simulink model "Bixler"  (R2018b)
settings: Solver=FixedStepAuto  StartTime=0.0  StopTime=inf  RelTol=1e-3
undefined symbols (not defined in the file or in its folder): dev, Main, pwm_output0
libraries: px4uORBlib x3, px4Sensorslib x2, simulink x2, px4lib x1, sharedtransform x1
settings Model: SimulationMode=external  ExtModeTrigDuration=10  Creator=Robert  LastModifiedBy=Robert
settings SolverCC: PositivePriorityOrder=on
settings OptimizationCC: EnhancedBackFolding=on  PassReuseOutputArgsAs=Individual arguments  MaxStackSize=64  OptimizeBlockOrder=speed  DifferentSizesBufferReuse=on  OptimizationCustomize=off
settings DebuggingCC: ParameterTunabilityLossMsg=error
settings HardwareCC: ProdBitPerPointer=32  ProdBitPerSizeT=32  ProdBitPerPtrDiffT=32  ProdLargestAtomicInteger=Long  ProdLargestAtomicFloat=Double  ProdWordSize=32  ProdLongLongMode=on  ProdHWDeviceType=ARM Compatible->ARM Cortex
settings SFSimCC: MATLABDynamicMemAlloc=off
settings RTWCC: SystemTargetFile=ert.tlc  HardwareBoard=PX4 Pixhawk 1  TLCOptions="-aInlineSetEventsForThisBaseRateFcn=TLC_FALSE -aSuppressMultiTaskScheduler=TLC_FALSE  -aRateBasedStepFcn=0"  TemplateMakefile=ert_default_tmf  GenerateReport=on  Toolchain=GNU Tools for PX4 Autopilots  IncludeHyperlinkInReport=on  LaunchReport=on  TargetLang=C++  GenerateTraceInfo=on  GenerateTraceReport=on  GenerateTraceReportSl=on  GenerateTraceReportSf=on  GenerateTraceReportEml=on
settings CodeAppCC: ForceParamTrailComments=on  IgnoreCustomStorageClasses=off  OperatorAnnotations=on  SimulinkDataObjDesc=on  SFDataObjDesc=on  InsertBlockDesc=on
settings ERTTargetCC: ExtMode=on  ExtModeMexArgs='127.0.0.1' 1 17725

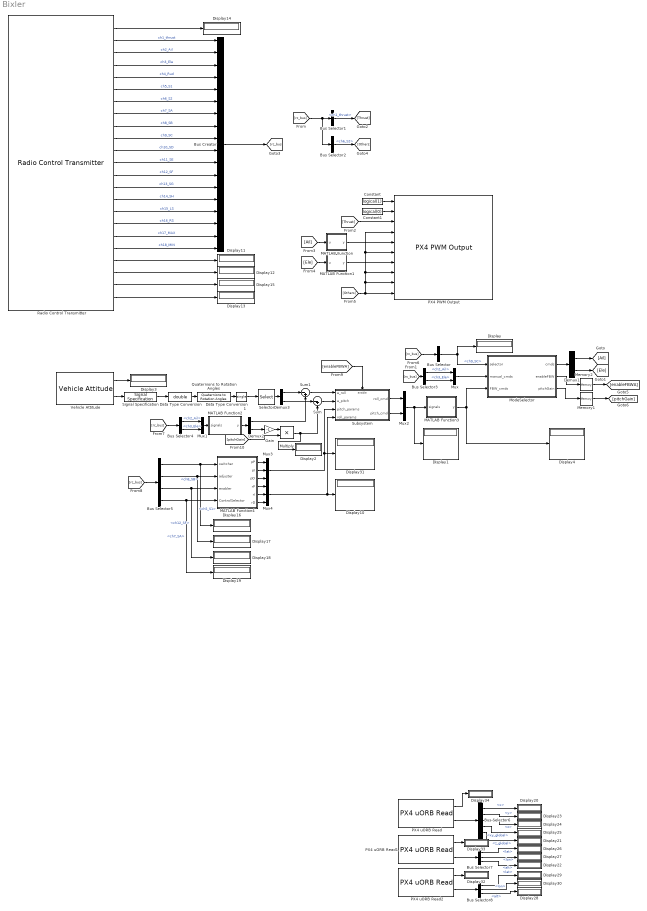
== system Bixler ==
  Bus Creator : BusCreator  Inputs=18
  Bus Selector : BusSelector  OutputSignals=ch9_SC
  Bus Selector1 : BusSelector  OutputSignals=ch1_thrust
  Bus Selector2 : BusSelector  OutputSignals=ch6_S2
  Bus Selector3 : BusSelector  OutputSignals=ch2_Ail,ch3_Ele
  Bus Selector4 : BusSelector  OutputSignals=ch2_Ail,ch3_Ele
  Bus Selector5 : BusSelector  OutputSignals=ch8_SB,ch5_S1,ch12_SF,ch7_SA
  Bus Selector6 : BusSelector  OutputSignals=x,y,z,xy_global,z_global
  Bus Selector7 : BusSelector  OutputSignals=lat,lon,alt
  Bus Selector8 : BusSelector  OutputSignals=lat,lon,alt
  Constant : Constant  Value=logical(1)
  Constant1 : Constant  Value=logical(0)
  Data Type Conversion : DataTypeConversion  OutDataTypeStr=double
  Data Type Conversion1 : DataTypeConversion  OutDataTypeStr=single
  Demux1 : Demux  Outputs=2
  Demux2 : Demux  Outputs=2
  Demux3 : Demux  Outputs=2
  Display{,1..4,10..34} (30 alike) : Display
  Gain : Gain  Gain=-1
  MATLAB Function : MATLAB Function  TreatAsAtomicUnit=on
  MATLAB Function1 : MATLAB Function  TreatAsAtomicUnit=on
  MATLAB Function2 : MATLAB Function  TreatAsAtomicUnit=on
  MATLAB Function3 : MATLAB Function  TreatAsAtomicUnit=on
  MATLAB Function4 : MATLAB Function  TreatAsAtomicUnit=on
  Memory1 : Memory
  Memory2 : Memory
  ModeSelector : MATLAB Function  TreatAsAtomicUnit=on
  Multiply : Product
  Mux : Mux  Inputs=2
  Mux1 : Mux  Inputs=2
  Mux2 : Mux  Inputs=2
  Mux3 : Mux  Inputs=3
  Mux4 : Mux  Inputs=3
  PX4 PWM Output : px4lib/PX4 PWM Output  pwmDevice=Main (/dev/pwm_output0)  pwmChannel1_=on  pwmChannel2_=on  pwmChannel3_=on  pwmChannel4_=on  pwmChannel5_=on  pwmChannel6_=on  pwmChannel7_=on  pwmChannel8_=on  forceTerminateFailsafe=off  outputErrorStatus=off
      settings: SourceProductName=Embedded Coder Support Package for PX4 Autopilots
  PX4 uORB Read : px4uORBlib/PX4 uORB Read  uORBTopic=vehicle_local_position  sampleTime=0.001  BlockingMode=off  BlockTimeout=1e-3
      settings: SourceProductName=Embedded Coder Support Package for PX4 Autopilots
  PX4 uORB Read1 : px4uORBlib/PX4 uORB Read  uORBTopic=vehicle_global_position  sampleTime=0.001  BlockingMode=off  BlockTimeout=1e-3
      settings: SourceProductName=Embedded Coder Support Package for PX4 Autopilots
  PX4 uORB Read2 : px4uORBlib/PX4 uORB Read  uORBTopic=vehicle_gps_position  sampleTime=0.001  BlockingMode=off  BlockTimeout=1e-3
      settings: SourceProductName=Embedded Coder Support Package for PX4 Autopilots
  Quaternions to Rotation Angles : sharedtransform/Quaternions to Rotation Angles  rotationOrder=ZYX  aMode=aMode
      settings: SourceProductBaseCode=AE
  Radio Control Transmitter : px4Sensorslib/Radio Control Transmitter  channel1=on  channel2=on  channel3=on  channel4=on  channel5=on  channel6=on  channel7=on  channel8=on  channel9=on  channel10=on  channel11=on  channel12=on  channel13=on  channel14=on  channel15=on  channel16=on  channel17=on  channel18=on  channel_count=on  rssi=on  rc_input_source=on  timestamp_last_signal=on  time_stamp=off  sampleTime=1/250  BlockingMode=off  BlockTimeout=5
      settings: SourceProductName=Embedded Coder Support Package for PX4 Autopilots
  Selector : Selector  InputPortWidth=3  IndexOptions=Index vector (dialog)  Indices=[3 2]  OutputSizes=1
  Signal Specification : SignalSpecification  OutDataTypeStr=single
  Subsystem : Subsystem
  Sum : Sum  Inputs=|-+
  Sum1 : Sum  Inputs=|-+
  Vehicle Attitude : px4Sensorslib/Vehicle Attitude  rollRate=off  pitchRate=off  yawRate=off  quaternion=on  uorbTimeStamp=off  BlockingMode=off  BlockTimeout=0.001  sampleTime=1/250
      settings: SourceProductName=Embedded Coder Support Package for PX4 Autopilots
  wires:
  Vehicle Attitude/2 -> Signal Specification/1
  Vehicle Attitude/1 -> Display3/1
  Radio Control Transmitter/8 -> Bus Creator/7  "ch7_SA"
  Radio Control Transmitter/7 -> Bus Creator/6  "ch6_S2"
  Radio Control Transmitter/6 -> Bus Creator/5  "ch5_S1"
  Radio Control Transmitter/2 -> Bus Creator/1  "ch1_thrust"
  Radio Control Transmitter/3 -> Bus Creator/2  "ch2_Ail"
  Radio Control Transmitter/4 -> Bus Creator/3  "ch3_Ele"
  Radio Control Transmitter/5 -> Bus Creator/4  "ch4_Rud"
  Radio Control Transmitter/9 -> Bus Creator/8  "ch8_SB"
  Radio Control Transmitter/20 -> Display11/1
  Radio Control Transmitter/21 -> Display12/1
  Radio Control Transmitter/23 -> Display13/1
  Radio Control Transmitter/1 -> Display14/1
  Radio Control Transmitter/22 -> Display15/1
  Constant/1 -> PX4 PWM Output/1
  Bus Selector1/1 -> [Thrust]  "<ch1_thrust>"
  [Others] -> PX4 PWM Output/6, PX4 PWM Output/4, PX4 PWM Output/8, PX4 PWM Output/9, PX4 PWM Output/10
  Constant1/1 -> PX4 PWM Output/2
  Bus Creator/1 -> [rc_bus]
  Quaternions to Rotation Angles/1 -> Data Type Conversion1/1
  Bus Selector/1 -> ModeSelector/1(selector), Display/1  "<ch9_SC>"
  Demux3/1 -> Sum1/1
  Demux3/2 -> Sum/1
  Mux2/1 -> Display1/1, MATLAB Function3/1(signals)
  Signal Specification/1 -> Data Type Conversion/1
  Data Type Conversion1/1 -> Selector/1
  [rc_bus] -> Bus Selector2/1, Bus Selector1/1
  [Thrust] -> PX4 PWM Output/3
  [Ail] -> MATLAB Function/1(u)
  [Ele] -> MATLAB Function1/1(u)
  [rc_bus] -> Bus Selector3/1
  [rc_bus] -> Bus Selector/1
  MATLAB Function3/1(y) -> ModeSelector/3(FBW_cmds), Display4/1
  Bus Selector3/1 -> Mux/1  "<ch2_Ail>"
  Bus Selector3/2 -> Mux/2  "<ch3_Ele>"
  Mux/1 -> ModeSelector/2(manual_cmds)
  ModeSelector/1(cmds) -> Demux1/1
  Demux1/1 -> [Ail]
  Demux1/2 -> [Ele]
  Bus Selector2/1 -> [Others]  "<ch6_S2>"
  Data Type Conversion/1 -> Quaternions to Rotation Angles/1
  MATLAB Function/1(y) -> PX4 PWM Output/5
  MATLAB Function1/1(y) -> PX4 PWM Output/7
  Demux2/2 -> Gain/1
  [rc_bus] -> Bus Selector4/1
  Bus Selector4/1 -> Mux1/1  "<ch2_Ail>"
  Bus Selector4/2 -> Mux1/2  "<ch3_Ele>"
  Mux1/1 -> MATLAB Function2/1(signals)
  MATLAB Function2/1(y) -> Demux2/1
  Demux2/1 -> Sum1/2
  Mux4/1 -> Subsystem/4(roll_params), Display10/1
  [rc_bus] -> Bus Selector5/1
  Bus Selector5/2 -> Display17/1, MATLAB Function4/2(adjuster)  "<ch5_S1>"
  Bus Selector5/1 -> Display16/1, MATLAB Function4/1(switcher)  "<ch8_SB>"
  MATLAB Function4/1(pP) -> Mux3/1
  MATLAB Function4/2(pI) -> Mux3/2
  MATLAB Function4/3(pD) -> Mux3/3
  Bus Selector5/3 -> Display18/1, MATLAB Function4/3(enabler)  "<ch12_SF>"
  Radio Control Transmitter/10 -> Bus Creator/9  "ch9_SC"
  Radio Control Transmitter/11 -> Bus Creator/10  "ch10_SD"
  Radio Control Transmitter/12 -> Bus Creator/11  "ch11_SE"
  Radio Control Transmitter/13 -> Bus Creator/12  "ch12_SF"
  Radio Control Transmitter/14 -> Bus Creator/13  "ch13_SG"
  Radio Control Transmitter/15 -> Bus Creator/14  "ch14_SH"
  Radio Control Transmitter/16 -> Bus Creator/15  "ch15_LS"
  Radio Control Transmitter/17 -> Bus Creator/16  "ch16_RS"
  Radio Control Transmitter/18 -> Bus Creator/17  "ch17_MAX"
  Radio Control Transmitter/19 -> Bus Creator/18  "ch18_MIN"
  MATLAB Function4/4(rP) -> Mux4/1
  MATLAB Function4/5(rI) -> Mux4/2
  MATLAB Function4/6(rD) -> Mux4/3
  Bus Selector5/4 -> Display19/1, MATLAB Function4/4(ControlSelector)  "<ch7_SA>"
  PX4 uORB Read/2 -> Bus Selector6/1
  PX4 uORB Read1/2 -> Bus Selector7/1
  PX4 uORB Read2/2 -> Bus Selector8/1
  PX4 uORB Read/1 -> Display34/1
  PX4 uORB Read1/1 -> Display33/1
  PX4 uORB Read2/1 -> Display32/1
  Bus Selector6/1 -> Display20/1  "<x>"
  Bus Selector6/2 -> Display23/1  "<y>"
  Bus Selector6/3 -> Display24/1  "<z>"
  Bus Selector6/4 -> Display25/1  "<xy_global>"
  Bus Selector6/5 -> Display21/1  "<z_global>"
  Bus Selector7/1 -> Display26/1  "<lat>"
  Bus Selector7/2 -> Display27/1  "<lon>"
  Bus Selector7/3 -> Display22/1  "<alt>"
  Bus Selector8/1 -> Display29/1  "<lat>"
  Bus Selector8/2 -> Display30/1  "<lon>"
  Bus Selector8/3 -> Display28/1  "<alt>"
  Sum1/1 -> Subsystem/1(e_roll)
  Sum/1 -> Subsystem/2(e_pitch)
  Subsystem/1(roll_cmd) -> Mux2/1
  Subsystem/2(pitch_cmd) -> Mux2/2
  [enableFBWA] -> Subsystem/Enable
  Multiply/1 -> Display2/1, Sum/2
  Mux3/1 -> Subsystem/3(pitch_params), Display31/1
  ModeSelector/2(enableFBW) -> Memory2/1
  Selector/1 -> Demux3/1
  Gain/1 -> Multiply/1
  ModeSelector/3(pitchGain) -> Memory1/1
  [pitchGain] -> Multiply/2
  Memory1/1 -> [pitchGain]
  Memory2/1 -> [enableFBWA]

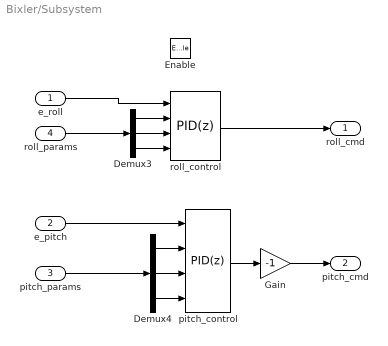
== system Bixler/Subsystem ==
  e_roll : Inport
  e_pitch : Inport  Port=2
  pitch_params : Inport  Port=3
  roll_params : Inport  Port=4
  Enable : EnablePort
  Demux3 : Demux  Outputs=3
  Demux4 : Demux  Outputs=3
  Gain : Gain  Gain=-1
  pitch_control : simulink/Continuous/PID Controller  Controller=PID  Form=Parallel  TimeDomain=Discrete-time  SampleTime=1/250  IntegratorMethod=Backward Euler  FilterMethod=Forward Euler  ControllerParametersSource=external  P=1  I=0  D=0  UseFilter=off  N=100  TunerSelectOption=Transfer Function Based (PID Tuner App)  InitialConditionSource=internal  InitialConditionForIntegrator=0  InitialConditionForFilter=0  DifferentiatorICPrevScaledInput=0  ExternalReset=none  TrackingMode=off  Kt=1  LimitOutput=on  UpperSaturationLimit=1  LowerSaturationLimit=-1  LinearizeAsGain=off  AntiWindupMode=clamping  Kb=1  PGainOutDataTypeStr=single  PProdOutDataTypeStr=single  POutMin=[]  POutMax=[]  IGainOutDataTypeStr=single  IProdOutDataTypeStr=single  IOutMin=[]  IOutMax=[]  DGainOutDataTypeStr=single  DProdOutDataTypeStr=single  DOutMin=[]  DOutMax=[]  NOutMin=[]  NOutMax=[]  SumOutDataTypeStr=single  SumOutMin=[]  SumOutMax=[]  SaturationOutDataTypeStr=single  SaturationOutMin=[]  SaturationOutMax=[]  PParamDataTypeStr=single  PParamMin=[]  PParamMax=[]  IParamDataTypeStr=single  IParamMin=[]  IParamMax=[]  DParamDataTypeStr=single  DParamMin=[]  DParamMax=[]  NParamMin=[]  NParamMax=[]  KbParamMin=[]  KbParamMax=[]  KtParamMin=[]  KtParamMax=[]  KbOutMin=[]  KbOutMax=[]  KtOutMin=[]  KtOutMax=[]  IntegratorOutDataTypeStr=single  IntegratorOutMin=[]  IntegratorOutMax=[]  FilterOutMin=[]  FilterOutMax=[]  SumI1OutMin=[]  SumI1OutMax=[]  SumI2OutMin=[]  SumI2OutMax=[]  SumI3OutMin=[]  SumI3OutMax=[]  SumI4OutMin=[]  SumI4OutMax=[]  SumDOutMin=[]  SumDOutMax=[]  SumAccumDataTypeStr=single  DifferentiatorOutDataTypeStr=single  DifferentiatorOutMin=[]  DifferentiatorOutMax=[]  FilterDiffOutCoefMin=[]  FilterDiffOutCoefMax=[]  ReciprocalOutMin=[]  ReciprocalOutMax=[]  SumDenOutMin=[]  SumDenOutMax=[]  SumNumOutMin=[]  SumNumOutMax=[]  DivideOutMin=[]  DivideOutMax=[]  IntegratorContinuousStateAttributes=''  IntegratorStateMustResolveToSignalObject=off  IntegratorRTWStateStorageClass=Auto  FilterContinuousStateAttributes=''  FilterStateMustResolveToSignalObject=off  FilterRTWStateStorageClass=Auto  ParallelPVariant=ExternalParameters  IdealPVariant=Disabled  IVariant=ExternalParameters  DVariant=ExternalParameters  IntegratorVariant=Discrete  SatVariant=Enabled  AWVariant=DiscClampingParallel  PCopyVariant=Disabled  TRVariant=Disabled  FdbkBlocksVariant=Feedback  IdealPFdbkVariant=Passthrough  SatFdbkVariant=Passthrough  DerivativeFilterVariant=Differentiator  NVariant=Passthrough  NCopyVariant=Disabled_SignalSpec  FilterICVariant=InternalICsDifferentiator  IntegratorICVariant=InternalICs  ExternalResetVariant=Disabled  TRSumVariant=Passthrough  SumFdbkVariant=Enabled  SumVariant=Sum_PID
  roll_control : simulink/Continuous/PID Controller  Controller=PID  Form=Parallel  TimeDomain=Discrete-time  SampleTime=1/250  IntegratorMethod=Backward Euler  FilterMethod=Forward Euler  ControllerParametersSource=external  P=1  I=0  D=0  UseFilter=off  N=100  TunerSelectOption=Transfer Function Based (PID Tuner App)  InitialConditionSource=internal  InitialConditionForIntegrator=0  InitialConditionForFilter=0  DifferentiatorICPrevScaledInput=0  ExternalReset=none  TrackingMode=off  Kt=1  LimitOutput=on  UpperSaturationLimit=1  LowerSaturationLimit=-1  LinearizeAsGain=off  AntiWindupMode=clamping  Kb=1  PGainOutDataTypeStr=single  PProdOutDataTypeStr=single  POutMin=[]  POutMax=[]  IGainOutDataTypeStr=single  IProdOutDataTypeStr=single  IOutMin=[]  IOutMax=[]  DGainOutDataTypeStr=single  DProdOutDataTypeStr=single  DOutMin=[]  DOutMax=[]  NOutMin=[]  NOutMax=[]  SumOutDataTypeStr=single  SumOutMin=[]  SumOutMax=[]  SaturationOutDataTypeStr=single  SaturationOutMin=[]  SaturationOutMax=[]  PParamDataTypeStr=single  PParamMin=[]  PParamMax=[]  IParamDataTypeStr=single  IParamMin=[]  IParamMax=[]  DParamDataTypeStr=single  DParamMin=[]  DParamMax=[]  NParamMin=[]  NParamMax=[]  KbParamMin=[]  KbParamMax=[]  KtParamMin=[]  KtParamMax=[]  KbOutMin=[]  KbOutMax=[]  KtOutMin=[]  KtOutMax=[]  IntegratorOutDataTypeStr=single  IntegratorOutMin=[]  IntegratorOutMax=[]  FilterOutMin=[]  FilterOutMax=[]  SumI1OutMin=[]  SumI1OutMax=[]  SumI2OutMin=[]  SumI2OutMax=[]  SumI3OutMin=[]  SumI3OutMax=[]  SumI4OutMin=[]  SumI4OutMax=[]  SumDOutMin=[]  SumDOutMax=[]  SumAccumDataTypeStr=single  DifferentiatorOutDataTypeStr=single  DifferentiatorOutMin=[]  DifferentiatorOutMax=[]  FilterDiffOutCoefMin=[]  FilterDiffOutCoefMax=[]  ReciprocalOutMin=[]  ReciprocalOutMax=[]  SumDenOutMin=[]  SumDenOutMax=[]  SumNumOutMin=[]  SumNumOutMax=[]  DivideOutMin=[]  DivideOutMax=[]  IntegratorContinuousStateAttributes=''  IntegratorStateMustResolveToSignalObject=off  IntegratorRTWStateStorageClass=Auto  FilterContinuousStateAttributes=''  FilterStateMustResolveToSignalObject=off  FilterRTWStateStorageClass=Auto  ParallelPVariant=ExternalParameters  IdealPVariant=Disabled  IVariant=ExternalParameters  DVariant=ExternalParameters  IntegratorVariant=Discrete  SatVariant=Enabled  AWVariant=DiscClampingParallel  PCopyVariant=Disabled  TRVariant=Disabled  FdbkBlocksVariant=Feedback  IdealPFdbkVariant=Passthrough  SatFdbkVariant=Passthrough  DerivativeFilterVariant=Differentiator  NVariant=Passthrough  NCopyVariant=Disabled_SignalSpec  FilterICVariant=InternalICsDifferentiator  IntegratorICVariant=InternalICs  ExternalResetVariant=Disabled  TRSumVariant=Passthrough  SumFdbkVariant=Enabled  SumVariant=Sum_PID
  roll_cmd : Outport
  pitch_cmd : Outport  Port=2
  wires:
  roll_control/1 -> roll_cmd/1
  Demux4/3 -> pitch_control/4
  Demux4/2 -> pitch_control/3
  Demux4/1 -> pitch_control/2
  pitch_params/1 -> Demux4/1
  Demux3/3 -> roll_control/4
  Demux3/2 -> roll_control/3
  Demux3/1 -> roll_control/2
  pitch_control/1 -> Gain/1
  e_roll/1 -> roll_control/1
  e_pitch/1 -> pitch_control/1
  roll_params/1 -> Demux3/1
  Gain/1 -> pitch_cmd/1

== matlab function Bixler/MATLAB Function1 ==
  data: u input uint16; y output uint16
function y = invertpwm(u)

y = uint16(1500-(single(u)-1500));

== matlab function Bixler/MATLAB Function ==
  data: u input uint16; y output uint16
function y = invertpwm(u)

y = uint16(1500-(single(u)-1500));

== matlab function Bixler/MATLAB Function2 ==
  data: signals input uint16; y output single
function y = pwm2signal(signals)

y = single(signals);
% Shift to center
y = y-1500;
% Range is ~1000-2000, ie +-500, but in is +-1
y = y./500;

== matlab function Bixler/MATLAB Function3 ==
  data: signals input; y output uint16
function y = signal2pwm(signals)

y = zeros(size(signals)); % y is hard set to uint16


% Range is ~1000-2000, ie +-500, but in is +-1
signals = signals.*500;
% Shift to center PWM
signals = signals+1500;
y = uint16(signals);

== matlab function Bixler/MATLAB Function4 ==
  data: switcher input uint16; pP output single; adjuster input uint16; pI output single; pD output single; enabler input uint16; ControlSelector input uint16; rP output single; rI output single; rD output single
function [pP,pI,pD,rP,rI,rD] = fcn(switcher, adjuster, enabler, ControlSelector)

persistent pkP pkI pkD rkP rkI rkD;
if isempty(pkP)
    pkP = single(1);
end
if isempty(pkI)
    pkI = single(0.4);
end
if isempty(pkD)
    pkD = single(0.025);
end
if isempty(rkP)
    rkP = single(1);
end
if isempty(rkI)
    rkI = single(0.4);
end
if isempty(rkD)
    rkD = single(0.05);
end

if enabler>1500
    if ControlSelector < 1400 % Top, Roll controll
        if switcher < 1400 % Top, P
            rkP = 1+(single(adjuster)-1500)./500; 
        elseif switcher > 1600 % Bottom, D
            rkD = 0.05+0.05*(single(adjuster)-1500)./500;
        else
            rkI = 0.4+0.4*(single(adjuster)-1500)./500;
        end
    elseif ControlSelector < 1600 % Mid, Pitch control
        if switcher < 1400 % Top, P
            pkP = 1+(single(adjuster)-1500)./500; 
        elseif switcher > 1600 % Bottom, D
            pkD = 0.025+0.025*(single(adjuster)-1500)./500;
        else
            pkI = 0.4+0.4*(single(adjuster)-1500)./500;
        end
    else
        % No controller set here yet
    end
end

pP = pkP;
pI = pkI;
pD = pkD;
rP = rkP;
rI = rkI;
rD = rkD;

== matlab function Bixler/ModeSelector ==
  data: selector input uint16; cmds output uint16 size=[2,1]; manual_cmds input uint16; FBW_cmds input uint16; enableFBW output boolean; pitchGain output
function [cmds,enableFBW,pitchGain] = fcn(selector, manual_cmds, FBW_cmds)

pitchGain = 1;
if selector>1600 % Auto mode, stick down on remote
    cmds = FBW_cmds;
    enableFBW = true;
    pitchGain = 1;
elseif selector>1400% Midpoint, as I flew at MUST first time
    cmds = FBW_cmds;
    enableFBW = true;
    pitchGain = 1.2;
else
    cmds = manual_cmds; % As midpoint, but less pitch sensitive.
    enableFBW = false;
end
